simulink model "first_compensation_figure"  (Simulink 7.3)
settings: Solver=ode45  StartTime=0.0  StopTime=10.0  RelTol=1e-3
libraries: powerlib_extras x1
settings Model: Creator=VAIO  LastModifiedBy=VAIO

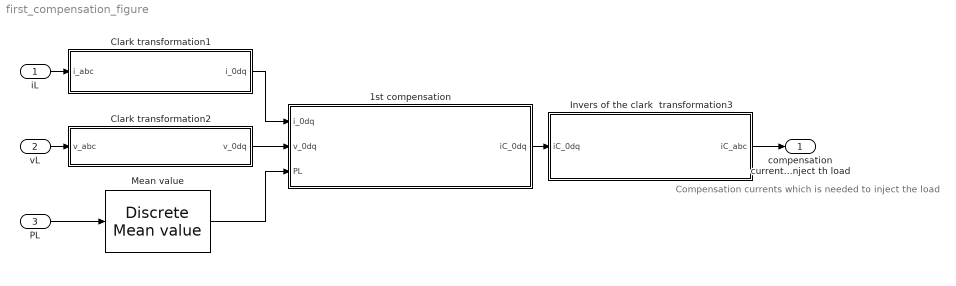
== system first_compensation_figure ==
  note: Compensation
      |  currents which is needed
      |  to inject the load
  iL : Inport  OutDataType=fixdt(1, 16)  OutScaling=2^0
  vL : Inport  Port=2  OutDataType=fixdt(1, 16)  OutScaling=2^0
  PL : Inport  Port=3  OutDataType=fixdt(1, 16)  OutScaling=2^0
  1st compensation : Stateflow chart  TreatAsAtomicUnit=on
  Clark transformation1 : Stateflow chart  TreatAsAtomicUnit=on
  Clark transformation2 : Stateflow chart  TreatAsAtomicUnit=on
  Invers of the clark  transformation3 : Stateflow chart  TreatAsAtomicUnit=on
  Mean value : powerlib_extras/Discrete Measurements/Discrete  Mean value  DialogController=POWERSYS.PowerSysDialog  SystemSampleTime=-1  Freq=50  Vinit=.001  Ts=50e-6
  compensation currents which is needed to inject th load : Outport  OutDataType=sfix(16)  OutScaling=2^0
  wires:
  Clark transformation1/1(i_0dq) -> 1st compensation/1(i_0dq)
  Clark transformation2/1(v_0dq) -> 1st compensation/2(v_0dq)
  Mean value/1 -> 1st compensation/3(PL)
  vL/1 -> Clark transformation2/1(v_abc)
  iL/1 -> Clark transformation1/1(i_abc)
  PL/1 -> Mean value/1
  1st compensation/1(iC_0dq) -> Invers of the clark  transformation3/1(iC_0dq)
  Invers of the clark  transformation3/1(iC_abc) -> compensation currents which is needed to inject th load/1

== matlab function Clark transformation1 ==
  data: i_abc input double; i_0dq output double
function i_0dq = mapping(i_abc)
%#eml

y =[1/sqrt(3) 1/sqrt(3) 1/sqrt(3); sqrt(2)/sqrt(3) -sqrt(2)/(2*sqrt(3)) -sqrt(2)/(2*sqrt(3)); 0 1/sqrt(2) -1/sqrt(2)]*a;

== matlab function Clark transformation2 ==
  data: v_abc input double; v_0dq output double
function v_0dq = mapping(v_abc)
%#eml

y =[1/sqrt(3) 1/sqrt(3) 1/sqrt(3); sqrt(2)/sqrt(3) -sqrt(2)/(2*sqrt(3)) -sqrt(2)/(2*sqrt(3)); 0 1/sqrt(2) -1/sqrt(2)]*a;

== matlab function 1st compensation ==
  data: i_0dq input double; v_0dq input double; PL input double; iC_0dq output double
function iC_0dq =  Vectorial_Method(i_0dq,v_0dq,PL)
%#eml

y =[1/sqrt(3) 1/sqrt(3) 1/sqrt(3); sqrt(2)/sqrt(3) -sqrt(2)/(2*sqrt(3)) -sqrt(2)/(2*sqrt(3)); 0 1/sqrt(2) -1/sqrt(2)]*a;

== matlab function Invers of the clark transformation3 ==
  data: iC_abc output double; iC_0dq input double
function iC_abc = mapping(iC_0dq)
%#eml

y =[1/sqrt(3) 1/sqrt(3) 1/sqrt(3); sqrt(2)/sqrt(3) -sqrt(2)/(2*sqrt(3)) -sqrt(2)/(2*sqrt(3)); 0 1/sqrt(2) -1/sqrt(2)]*a;
